simulink model "FisherSimmons"  (R2016b)
settings: Solver=VariableStepAuto  StartTime=0.0  StopTime=10.0  RelTol=1e-3
libraries: simulink x3
settings Model: Creator=charAn  LastModifiedBy=charAn

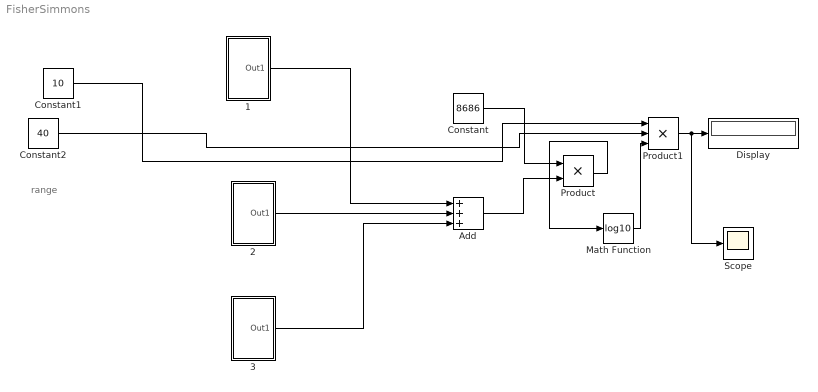
== system FisherSimmons ==
  note: range
  "1 " : Subsystem
  2 : Subsystem
  "3 " : Subsystem
  Add : Sum  Inputs=+++
  Constant : Constant  Value=8686
  Constant1 : Constant  Value=10
  Constant2 : Constant  Value=40
  Display : Display
  Math Function : Math  Operator=log10  SaturateOnIntegerOverflow=on
  Product : Product
  Product1 : Product  Inputs=3
  Scope : Scope
  wires:
  "1 "/1(Out1) -> Add/1
  2/1(Out1) -> Add/2
  "3 "/1(Out1) -> Add/3
  Constant/1 -> Product/1
  Add/1 -> Product/2
  Constant1/1 -> Product1/1
  Product/1 -> Math Function/1
  Constant2/1 -> Product1/2
  Math Function/1 -> Product1/3
  Product1/1 -> Scope/1, Display/1

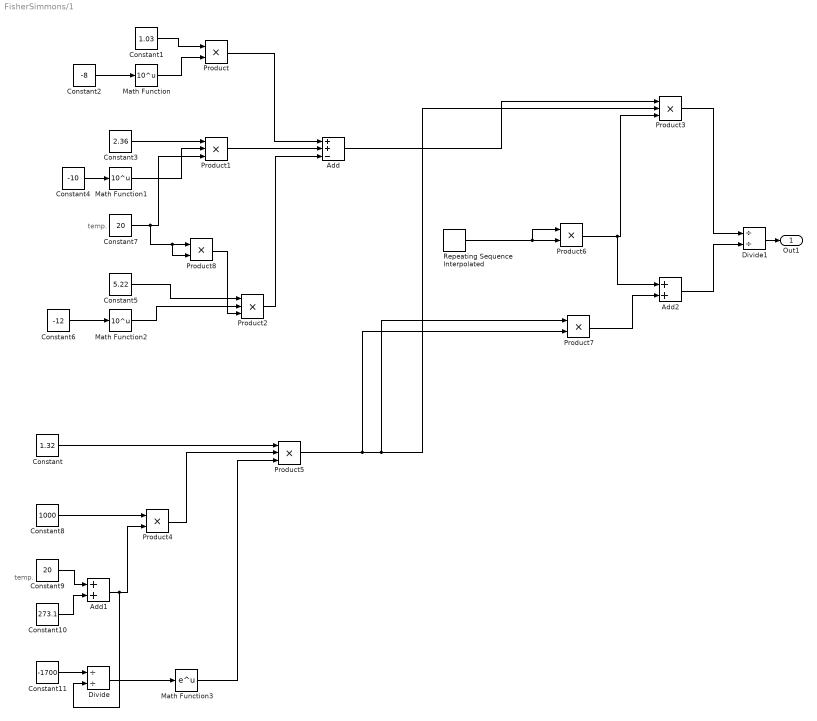
== system FisherSimmons/1  ==
  note: temp.
  note: temp.
  Add : Sum  Inputs=++-
  Add1 : Sum
  Add2 : Sum
  Constant : Constant  Value=1.32
  Constant1 : Constant  Value=1.03
  Constant10 : Constant  Value=273.1
  Constant11 : Constant  Value=-1700
  Constant2 : Constant  Value=-8
  Constant3 : Constant  Value=2.36
  Constant4 : Constant  Value=-10
  Constant5 : Constant  Value=5.22
  Constant6 : Constant  Value=-12
  Constant7 : Constant  Value=20
  Constant8 : Constant  Value=1000
  Constant9 : Constant  Value=20
  Divide : Product  Inputs=//
  Divide1 : Product  Inputs=//
  Math Function : Math  Operator=10^u  SaturateOnIntegerOverflow=on
  Math Function1 : Math  Operator=10^u  SaturateOnIntegerOverflow=on
  Math Function2 : Math  Operator=10^u  SaturateOnIntegerOverflow=on
  Math Function3 : Math  SaturateOnIntegerOverflow=on
  Product{,4,6..8} (5 alike) : Product
  Product{1..3,5} (4 alike) : Product  Inputs=3
  Repeating Sequence Interpolated : simulink/Sources/Repeating Sequence Interpolated  OutValues=[0 1000 2000 3000 4000 5000 6000 7000 8000 9000 10000]  TimeValues=[0 10 20 30 40 50 60 70 80 90 100]  LookUpMeth=Interpolation-Use End Values  tsamp=0.01  OutMin=[]  OutMax=[]  OutDataTypeStr=double  OutputDataTypeScalingMode=double  OutDataType=fixdt(0,8)  OutScaling=2^-10
  Out1 : Outport
  wires:
  Product1/1 -> Add/2
  Constant4/1 -> Math Function1/1
  Constant11/1 -> Divide/1
  Math Function/1 -> Product/2
  Constant6/1 -> Math Function2/1
  Constant9/1 -> Add1/1
  Add/1 -> Product3/1
  Constant/1 -> Product5/1
  Constant8/1 -> Product4/1
  Product/1 -> Add/1
  Add1/1 -> Divide/2, Product4/2
  Product3/1 -> Divide1/1
  Product2/1 -> Add/3
  Product7/1 -> Add2/2
  Product5/1 -> Product7/2, Product7/1, Product3/2
  Product6/1 -> Add2/1, Product3/3
  Divide1/1 -> Out1/1
  Repeating Sequence Interpolated/1 -> Product6/1, Product6/2
  Math Function1/1 -> Product1/2
  Constant3/1 -> Product1/1
  Constant5/1 -> Product2/1
  Add2/1 -> Divide1/2
  Divide/1 -> Math Function3/1
  Math Function3/1 -> Product5/3
  Constant1/1 -> Product/1
  Constant10/1 -> Add1/2
  Math Function2/1 -> Product2/2
  Constant7/1 -> Product8/2, Product8/1, Product1/3
  Product4/1 -> Product5/2
  Constant2/1 -> Math Function/1
  Product8/1 -> Product2/3

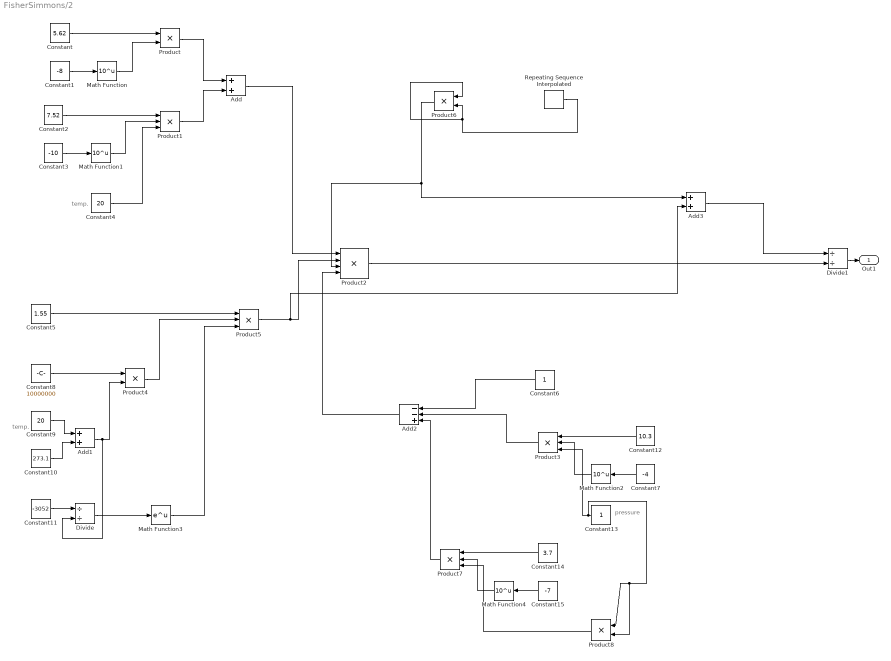
== system FisherSimmons/2 ==
  note: pressure
  note: temp.
  note: temp.
  Add : Sum
  Add1 : Sum
  Add2 : Sum  Inputs=--+
  Add3 : Sum
  Constant : Constant  Value=5.62
  Constant1 : Constant  Value=-8
  Constant10 : Constant  Value=273.1
  Constant11 : Constant  Value=-3052
  Constant12 : Constant  Value=10.3
  Constant13 : Constant
  Constant14 : Constant  Value=3.7
  Constant15 : Constant  Value=-7
  Constant2 : Constant  Value=7.52
  Constant3 : Constant  Value=-10
  Constant4 : Constant  Value=20
  Constant5 : Constant  Value=1.55
  Constant6 : Constant
  Constant7 : Constant  Value=-4
  Constant8 : Constant  Value=10000000
  Constant9 : Constant  Value=20
  Divide : Product  Inputs=//
  Divide1 : Product  Inputs=//
  Math Function{,1..2,4} (4 alike) : Math  Operator=10^u  SaturateOnIntegerOverflow=on
  Math Function3 : Math  SaturateOnIntegerOverflow=on
  Product{,4,6,8} (4 alike) : Product
  Product{1,3,5,7} (4 alike) : Product  Inputs=3
  Product2 : Product  Inputs=4
  Repeating Sequence Interpolated : simulink/Sources/Repeating Sequence Interpolated  OutValues=[0 1000 2000 3000 4000 5000 6000 7000 8000 9000 10000]  TimeValues=[0 10 20 30 40 50 60 70 80 90 100]  LookUpMeth=Interpolation-Use End Values  tsamp=0.01  OutMin=[]  OutMax=[]  OutDataTypeStr=double  OutputDataTypeScalingMode=double  OutDataType=fixdt(0,8)  OutScaling=2^-10
  Out1 : Outport
  wires:
  Add1/1 -> Divide/2, Product4/2
  Constant1/1 -> Math Function/1
  Divide1/1 -> Out1/1
  Constant14/1 -> Product7/1
  Add/1 -> Product2/1
  Product/1 -> Add/1
  Constant3/1 -> Math Function1/1
  Constant2/1 -> Product1/1
  Math Function1/1 -> Product1/2
  Constant/1 -> Product/1
  Constant8/1 -> Product4/1
  Product1/1 -> Add/2
  Product6/1 -> Add3/1, Product2/3
  Constant4/1 -> Product1/3
  Repeating Sequence Interpolated/1 -> Product6/1, Product6/2
  Constant13/1 -> Product8/2, Product8/1, Product3/3
  Constant15/1 -> Math Function4/1
  Math Function2/1 -> Product3/2
  Constant6/1 -> Add2/1
  Product8/1 -> Product7/3
  Constant12/1 -> Product3/1
  Product3/1 -> Add2/2
  Constant7/1 -> Math Function2/1
  Product2/1 -> Divide1/2
  Add2/1 -> Product2/4
  Product7/1 -> Add2/3
  Constant5/1 -> Product5/1
  Constant10/1 -> Add1/2
  Constant9/1 -> Add1/1
  Math Function/1 -> Product/2
  Product4/1 -> Product5/2
  Product5/1 -> Add3/2, Product2/2
  Math Function4/1 -> Product7/2
  Math Function3/1 -> Product5/3
  Constant11/1 -> Divide/1
  Divide/1 -> Math Function3/1
  Add3/1 -> Divide1/1

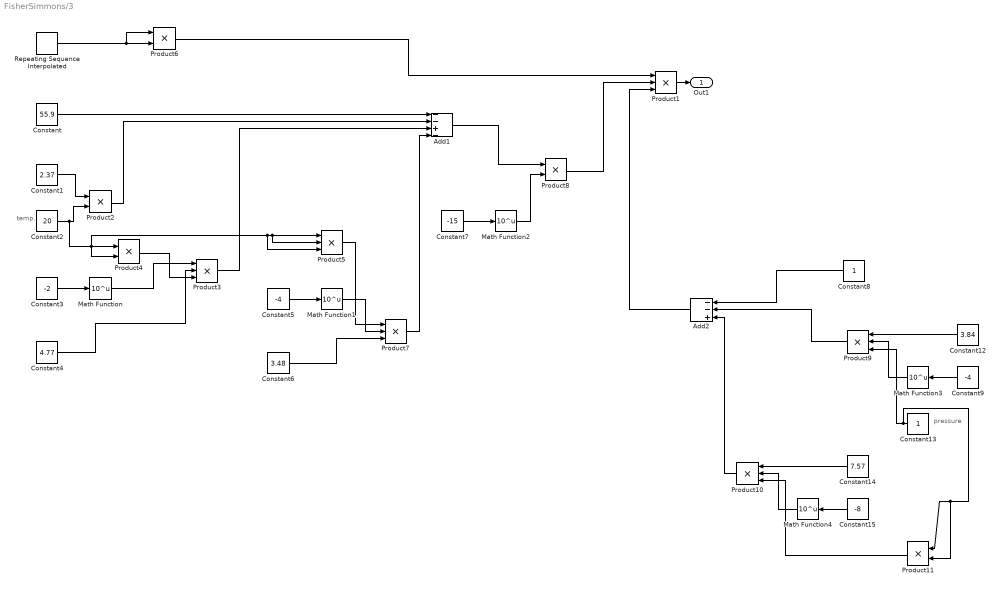
== system FisherSimmons/3  ==
  note: temp.
  note: pressure
  Add1 : Sum  Inputs=--+-
  Add2 : Sum  Inputs=--+
  Constant : Constant  Value=55.9
  Constant1 : Constant  Value=2.37
  Constant12 : Constant  Value=3.84
  Constant13 : Constant
  Constant14 : Constant  Value=7.57
  Constant15 : Constant  Value=-8
  Constant2 : Constant  Value=20
  Constant3 : Constant  Value=-2
  Constant4 : Constant  Value=4.77
  Constant5 : Constant  Value=-4
  Constant6 : Constant  Value=3.48
  Constant7 : Constant  Value=-15
  Constant8 : Constant
  Constant9 : Constant  Value=-4
  Math Function{,1..4} (5 alike) : Math  Operator=10^u  SaturateOnIntegerOverflow=on
  Product{1,3,5,7,9..10} (6 alike) : Product  Inputs=3
  Product{2,4,6,8,11} (5 alike) : Product
  Repeating Sequence Interpolated : simulink/Sources/Repeating Sequence Interpolated  OutValues=[0 1000 2000 3000 4000 5000 6000 7000 8000 9000 10000]  TimeValues=[0 10 20 30 40 50 60 70 80 90 100]  LookUpMeth=Interpolation-Use End Values  tsamp=0.01  OutMin=[]  OutMax=[]  OutDataTypeStr=double  OutputDataTypeScalingMode=double  OutDataType=fixdt(0,8)  OutScaling=2^-10
  Out1 : Outport
  wires:
  Constant/1 -> Add1/1
  Product2/1 -> Add1/2
  Constant1/1 -> Product2/1
  Product4/1 -> Product3/3
  Math Function/1 -> Product3/1
  Constant4/1 -> Product3/2
  Product7/1 -> Add1/4
  Product3/1 -> Add1/3
  Constant7/1 -> Math Function2/1
  Constant5/1 -> Math Function1/1
  Add1/1 -> Product8/1
  Constant6/1 -> Product7/3
  Product9/1 -> Add2/2
  Constant8/1 -> Add2/1
  Math Function2/1 -> Product8/2
  Product8/1 -> Product1/2
  Add2/1 -> Product1/3
  Product1/1 -> Out1/1
  Repeating Sequence Interpolated/1 -> Product6/1, Product6/2
  Product5/1 -> Product7/1
  Constant2/1 -> Product5/3, Product5/2, Product5/1, Product4/2, Product4/1, Product2/2
  Math Function1/1 -> Product7/2
  Product6/1 -> Product1/1
  Constant3/1 -> Math Function/1
  Math Function3/1 -> Product9/2
  Constant13/1 -> Product11/2, Product11/1, Product9/3
  Constant15/1 -> Math Function4/1
  Math Function4/1 -> Product10/2
  Constant12/1 -> Product9/1
  Product11/1 -> Product10/3
  Product10/1 -> Add2/3
  Constant9/1 -> Math Function3/1
  Constant14/1 -> Product10/1
